simulink model "MDL_liniowy_nieliniowy_lead_lag"  (R2023a)
settings: Solver=ode4  StartTime=0.0  StopTime=end_time  FixedStep=dt  MaxStep=0.001  RelTol=1e-3
values from neighbouring files (symbols this model uses):
  A = [ ... (first row only)    [anim_sim_script.m]    (also in lin_nonlin_lead_lag.m)
  B = [0;0;b1;b2]    [anim_sim_script.m]    (also in lin_nonlin_lead_lag.m)
  H = series(lead, lag)    [anim_sim_script.m]    (also in lin_nonlin_lead_lag.m)
  IC = [x_ic, theta_ic, D_x_ic, D_theta_ic]'    [anim_sim_script.m]    (also in lin_nonlin_lead_lag.m)
  IClin = [x_ic, -delta_thetaIC*pi/180, 0, 0]    [anim_sim_script.m]    (also in lin_nonlin_lead_lag.m)
  K = 2    [lin_nonlin_lead_lag.m]
  Kx = 7.5    [lin_nonlin_lead_lag.m]
settings Model: Creator=Adam  LastModifiedBy=Adam
settings SolverCC: AlgebraicLoopSolver=TrustRegion
settings DataIOCC: SaveOutput=off  SignalLogging=off  DSMLogging=off
settings DebuggingCC: AlgebraicLoopMsg=none  UnconnectedInputMsg=warning  UnconnectedOutputMsg=warning  UnconnectedLineMsg=warning
settings ModelReferenceCC: EnableRefExpFcnMdlSchedulingChecks=on
settings RTWCC: DLArmComputeVersion=19.05

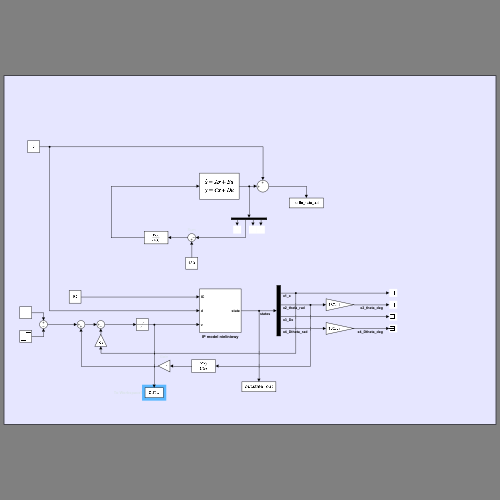
[thumbnail: Simulink's stored preview of the top-level diagram]
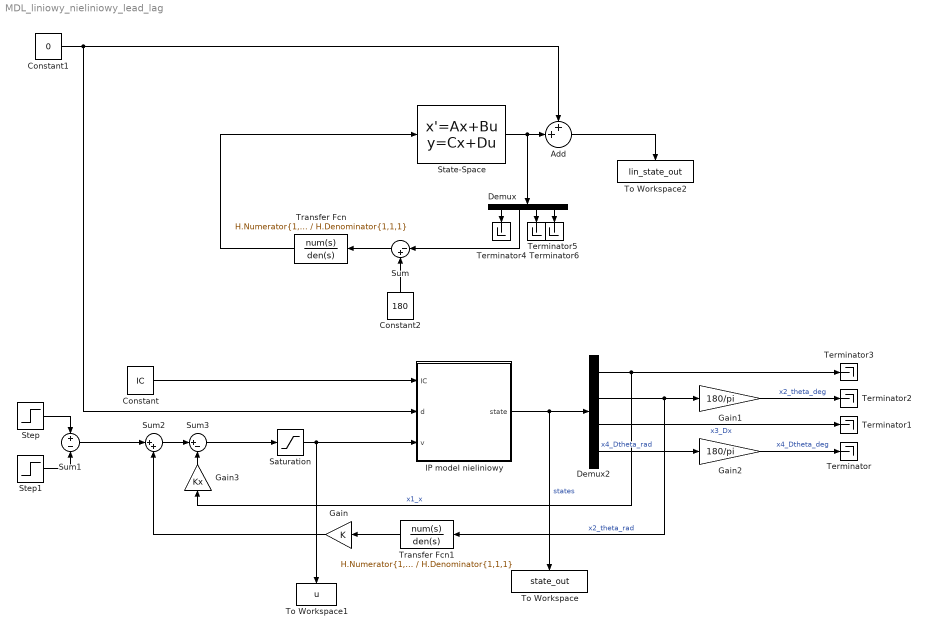
== system MDL_liniowy_nieliniowy_lead_lag ==
  Add : Sum  Inputs=++|
  Constant : Constant  Value=IC
  Constant1 : Constant  Value=0
  Constant2 : Constant  Value=180
  Demux : Demux
  Demux2 : Demux
  Gain : Gain  Gain=K
  Gain1 : Gain  Gain=180/pi
  Gain2 : Gain  Gain=180/pi
  Gain3 : Gain  Gain=Kx
  IP model nieliniowy : Subsystem
  Saturation : Saturate  UpperLimit=12  LowerLimit=-12
  State-Space : StateSpace  A=A  B=B  C=eye(4)  D=zeros([4 1])  InitialCondition=IClin
  Step : Step  Time=0  After=5  SampleTime=0
  Step1 : Step  Time=0.1  After=5  SampleTime=0
  Sum : Sum  Inputs=|-+
  Sum1 : Sum  Inputs=+-
  Sum2 : Sum  Inputs=|++
  Sum3 : Sum  Inputs=|+-
  Terminator{,1..6} (7 alike) : Terminator
  To Workspace : ToWorkspace  VariableName=state_out  SampleTime=-1
  To Workspace1 : ToWorkspace  VariableName=u  SampleTime=-1
  To Workspace2 : ToWorkspace  VariableName=lin_state_out  SampleTime=-1
  Transfer Fcn : TransferFcn  Numerator=H.Numerator{1,1,1}  Denominator=H.Denominator{1,1,1}
  Transfer Fcn1 : TransferFcn  Numerator=H.Numerator{1,1,1}  Denominator=H.Denominator{1,1,1}
  wires:
  Gain2/1 -> Terminator/1  "x4_Dtheta_deg"
  Demux2/4 -> Gain2/1  "x4_Dtheta_rad"
  Demux2/3 -> Terminator1/1  "x3_Dx"
  Demux2/2 -> Transfer Fcn1/1, Gain1/1  "x2_theta_rad"
  Demux2/1 -> Terminator3/1, Gain3/1  "x1_x"
  Gain1/1 -> Terminator2/1  "x2_theta_deg"
  IP model nieliniowy/1(state) -> Demux2/1, To Workspace/1  "states"
  Constant/1 -> IP model nieliniowy/1(IC)
  State-Space/1 -> Demux/1, Add/2
  Constant1/1 -> IP model nieliniowy/2(d), Add/1
  Add/1 -> To Workspace2/1
  Transfer Fcn/1 -> State-Space/1
  Demux/4 -> Terminator6/1
  Demux/3 -> Terminator5/1
  Demux/1 -> Terminator4/1
  Demux/2 -> Sum/1
  Sum/1 -> Transfer Fcn/1
  Constant2/1 -> Sum/2
  Transfer Fcn1/1 -> Gain/1
  Gain/1 -> Sum2/2
  Step/1 -> Sum1/1
  Step1/1 -> Sum1/2
  Sum1/1 -> Sum2/1
  Sum2/1 -> Sum3/1
  Sum3/1 -> Saturation/1
  Gain3/1 -> Sum3/2
  Saturation/1 -> To Workspace1/1, IP model nieliniowy/3(v)

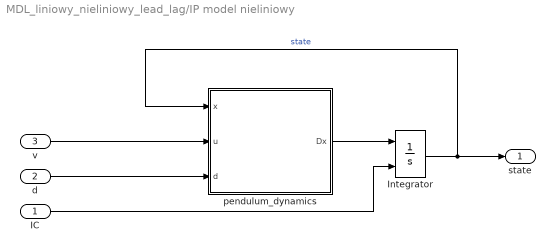
== system MDL_liniowy_nieliniowy_lead_lag/IP model nieliniowy ==
  IC : Inport
  d : Inport  Port=2
  v : Inport  Port=3
  Integrator : Integrator  InitialConditionSource=external
  pendulum_dynamics : MATLAB Function  TreatAsAtomicUnit=on
  state : Outport
  wires:
  Integrator/1 -> state/1, pendulum_dynamics/1(x)  "state"
  v/1 -> pendulum_dynamics/2(u)
  pendulum_dynamics/1(Dx) -> Integrator/1
  IC/1 -> Integrator/2
  d/1 -> pendulum_dynamics/3(d)

== matlab function MDL_liniowy_nieliniowy_lead_lag/IP model nieliniowy/pendulum_dynamics ==
  data: x input; u input; d input; Dx output; params_lepkie parameter
function Dx = dynamika_wahadla(x, u, d, params_lepkie)
% x : stan
% u : input - napięcie
%
% params scope: "parameters"
%

% State, function input: x = [x Dx theta Dtheta]'
x1 = x(1);
x2 = x(2); 
x3 = x(3);
x4 = x(4);

params_lepkie = num2cell(params_lepkie);
[M, mc, mp, Lp, Lc, g, b, gamma, mr, Mt, L, Jcm, Jt, alpha, beta] = params_lepkie{:};

% Equations for pendulum dynamics
Ff = b*x3;
Fi = alpha*u - beta*x3;
A = d*cos(x2) - Ff + L*mr*x4^2*sin(x2) + Fi;
B = d*Lc + L*g*mr*sin(x2) - gamma*x4;
DEN = Jt*Mt - (L*mr*cos(x2))^2;

ddt_x1 = x3;
ddt_x2 = x4;
ddt_x3 = (Jt*A - L*mr*cos(x2)*B) / DEN;
ddt_x4 = (Mt*B - L*mr*cos(x2)*A) / DEN;

% output
Dx = [ddt_x1 ddt_x2 ddt_x3 ddt_x4]';

end
